simulink model "F550_verify_trim"  (R2024a)
settings: Solver=VariableStepAuto  StartTime=0.0  StopTime=100  FixedStep=0.001  RelTol=1e-3
undefined symbols (not defined in the file): r2d, u0
settings Model: Creator=ADMIN  LastModifiedBy=CNU_UASG
settings DataIOCC: ExternalInput=getinputstruct(op_trim1)  InitialState=getstatestruct(op_trim1)
settings DebuggingCC: UnconnectedInputMsg=warning  UnconnectedOutputMsg=warning  UnconnectedLineMsg=warning
settings ModelReferenceCC: EnableRefExpFcnMdlSchedulingChecks=on
settings RTWCC: GPUComputeCapability=3.5  DLArmComputeVersion=19.05

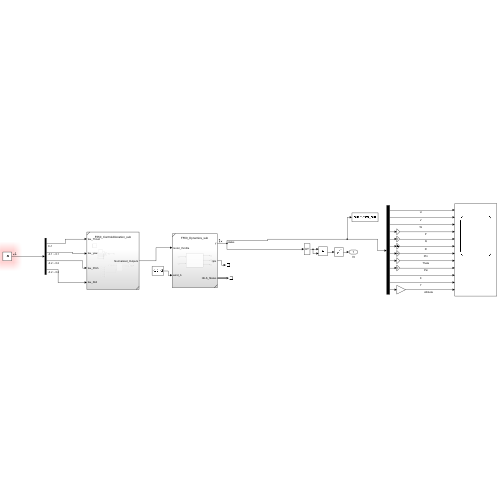
[thumbnail: Simulink's stored preview of the top-level diagram]
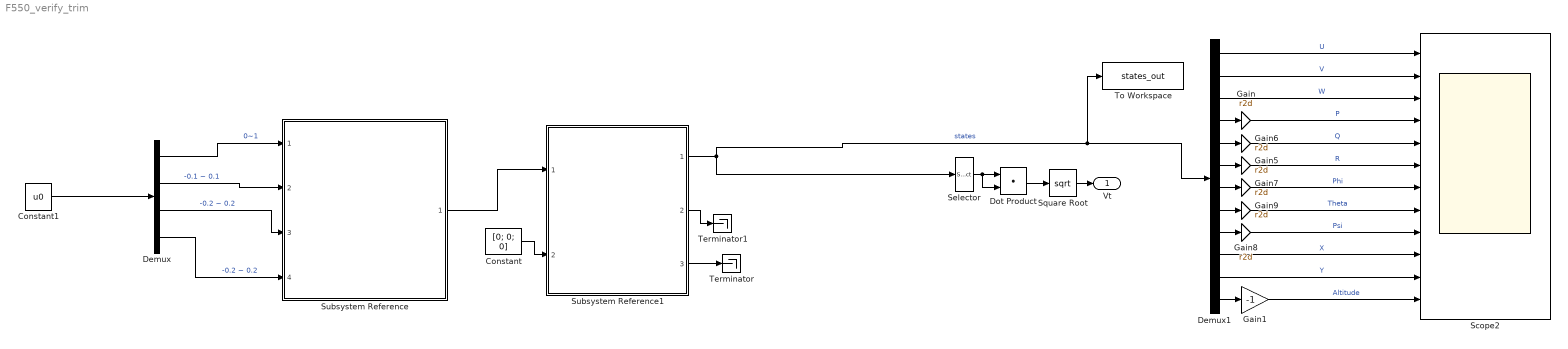
== system F550_verify_trim ==
  Constant : Constant  Value=[0; 0; 0]
  Constant1 : Constant  Value=u0
  Demux : Demux
  Demux1 : Demux  Outputs=12
  Dot Product : DotProduct  OutDataTypeStr=Inherit: Inherit via internal rule
  Gain{,5..9} (6 alike) : Gain  Gain=r2d
  Gain1 : Gain  Gain=-1
  Scope2 : Scope  NumInputPorts=12
  Selector : Selector  InputPortWidth=12  IndexOptions=Index vector (dialog)  Indices=[1 2 3]  OutputSizes=1
  Square Root : Sqrt
  Subsystem Reference : Subsystem  ReferencedSubsystem=F550_ControlAllocation_sub
  Subsystem Reference1 : Subsystem  ReferencedSubsystem=F550_Dynamics_sub
  Terminator : Terminator
  Terminator1 : Terminator
  To Workspace : ToWorkspace  VariableName=states_out  SampleTime=-1
  Vt : Outport
  wires:
  Demux/4 -> Subsystem Reference/4  "-0.2 ~ 0.2"
  Demux/3 -> Subsystem Reference/3  "-0.2 ~ 0.2"
  Demux/2 -> Subsystem Reference/2  "-0.1 ~ 0.1"
  Demux/1 -> Subsystem Reference/1  "0~1"
  Selector/1 -> Dot Product/1, Dot Product/2
  Square Root/1 -> Vt/1
  Dot Product/1 -> Square Root/1
  Subsystem Reference1/1 -> Demux1/1, To Workspace/1, Selector/1  "states"
  Subsystem Reference1/3 -> Terminator/1
  Constant/1 -> Subsystem Reference1/2
  Subsystem Reference/1 -> Subsystem Reference1/1
  Subsystem Reference1/2 -> Terminator1/1
  Gain5/1 -> Scope2/6  "R"
  Demux1/9 -> Gain8/1
  Demux1/7 -> Gain7/1
  Demux1/3 -> Scope2/3  "W"
  Demux1/1 -> Scope2/1  "U"
  Demux1/2 -> Scope2/2  "V"
  Demux1/4 -> Gain/1
  Gain8/1 -> Scope2/9  "Psi"
  Gain7/1 -> Scope2/7  "Phi"
  Demux1/8 -> Gain9/1
  Demux1/5 -> Gain6/1
  Gain/1 -> Scope2/4  "P"
  Gain6/1 -> Scope2/5  "Q"
  Gain9/1 -> Scope2/8  "Theta"
  Demux1/6 -> Gain5/1
  Demux1/10 -> Scope2/10  "X"
  Demux1/11 -> Scope2/11  "Y"
  Demux1/12 -> Gain1/1
  Gain1/1 -> Scope2/12  "Altitude"
  Constant1/1 -> Demux/1
